simulink model "flightControlSystem"  (R2024a)
settings: Solver=ode3  StartTime=0  StopTime=TFinal  FixedStep=Ts  RelTol=1e-3  EnableMultiTasking=on
model workspace (MAT data in the model file):
  CIRCLE_PTS = [19 19 19]
  ZEROS = [0 0 0 0 0 0 0 0 0 0 0 0 ... (1444 elements, 38x38)]
undefined symbols (not defined in the file): codertarget, Controller, DiscIntNeverNeededParam, Discrete, Estimator, g, gray, init, Sensors, Time, Ts, var_acc_angle_N, var_bias_gyr_N, var_gyro_p_N, Vehicle
libraries: simulink x38, slpidlib x4, ctrlSharedLib x4, sharedtransform x3, visiontextngfix x1, parrotlib x1
(part 3 of 3)

== matlab function flightControlSystem/Image Processing System/Subsystem2/Subsystem1/scan_range ==
  data: result output; u input; startX input; startY input; endX input; endY input; isScanning input
function result = scan_range(u, startX, startY, endX, endY, isScanning)

currentX = 1;
currentY = 2;
movementSpeed = 0;
redLinePresence = u(60, 80);

persistent previousEndlessX;
persistent previousEndlessY;

if isScanning
    if redLinePresence == 1  % ------ inside red-line ------
    
        maxDistance = 0;
        count = 0;

        endlessX = [0 0];
        endlessY = [0 0];
        timeCount = [0 0];

        isEndless = false;
        endlessIndex = 0;
        
        edgeDir = edgeCount(startX, startY);
        xi = startX;  yi = startY; direction = 1;
        
        if edgeDir == 1 || edgeDir == 4
            direction = -1;
        end
        
        while xi ~= endX || yi ~= endY
            distance = drawLine(60, 80, xi, yi, u, 0);

            if distance == 0 % if endless

                if ~isEndless
                    isEndless = true;
                    endlessIndex = endlessIndex + 1;
                end
                if endlessIndex > 2
                    break;
                end
                
                endlessX(endlessIndex) = endlessX(endlessIndex) + xi;
                endlessY(endlessIndex) = endlessY(endlessIndex) + yi;
                timeCount(endlessIndex) = timeCount(endlessIndex) + 1;

            else
                isEndless = false;
                if distance > maxDistance
                    maxDistance = distance;
                    currentX = xi; 
                    currentY = yi;
                    count = 1;
                end
            end

            % Iteration
            edgeDir = edgeCount(xi, yi);
            if edgeDir == 1 || edgeDir == 3
                yi = yi + direction;
            else
                xi = xi + direction;
            end
            if xi < 1
                yi = 159; xi = 1; direction = -1;
            elseif xi > 120
                xi = 120; yi = 2; direction = 1;
            elseif yi < 1
                yi = 1; xi = 2; direction = 1;
            elseif yi > 160
                yi = 160; xi = 119; direction = -1;
            end
        end % while end

        if endlessIndex == 1 % ---------- 1 endless ------------
            currentX = endlessX(1);
            currentY = endlessY(1);
            count = timeCount(1);

            currentX = round(currentX / count);
            currentY = round(currentY / count);
            [currentX, currentY] = closestEdge(currentX, currentY);

            previousEndlessX = 60 + (60 - currentX) + 1;
            previousEndlessY = 80 + (80 - currentY) + 1;

        elseif endlessIndex == 2 % ---------- 2 endless ------------
            
            if isempty(previousEndlessX)
                currentX = endlessX(1);
                currentY = endlessY(1);
                count = timeCount(1);
    
                currentX = round(currentX / count);
                currentY = round(currentY / count);
                [currentX, currentY] = closestEdge(currentX, currentY);
    
                previousEndlessX = 60 + (60 - currentX) + 1;
                previousEndlessY = 80 + (80 - currentY) + 1;
            else
                midPoints = [0 0; 0 0];
                for i = 1:2
                    x = endlessX(i);
                    y = endlessY(i);
                    t = timeCount(i);

                    x = round(x / t);
                    y = round(y / t);
                    
                    [x, y] = closestEdge(x, y);
                    
                    midPoints(i, 1) = x;
                    midPoints(i, 2) = y;
                end

                diff1X = previousEndlessX - midPoints(1, 1);
                diff1Y = previousEndlessY - midPoints(1, 2);
                diff2X = previousEndlessX - midPoints(2, 1);
                diff2Y = previousEndlessY - midPoints(2, 2);
                distance1 = sqrt(diff1X * diff1X + diff1Y * diff1Y);
                distance2 = sqrt(diff2X * diff2X + diff2Y * diff2Y);

                if distance1 > distance2
                    currentX = midPoints(1, 1);
                    currentY = midPoints(1, 2);
                else
                    currentX = midPoints(2, 1);
                    currentY = midPoints(2, 2);
                end
                
                previousEndlessX = 60 + (60 - currentX) + 1;
                previousEndlessY = 80 + (80 - currentY) + 1;
                
            end
        else % ---------- NO endless ------------
            movementSpeed = maxDistance;
        end

    else % ----------------- outside red line ----------------------
        startX = 2; startY = 1;
        endX = 1; endY = 1;
        
        MAX_DISTANCE = 100;
        minDistance = MAX_DISTANCE;
        edgeDir = edgeCount(startX, startY);
        xi = startX;  yi = startY; direction = 1;
        if edgeDir == 1 || edgeDir == 4
            direction = -1;
        end
        
        while xi ~= endX || yi ~= endY
            distance = drawLine(60, 80, xi, yi, u, 1);
    
            if distance > 0 && distance < minDistance
                minDistance = distance;
                currentX = xi;
                currentY = yi;
            end
    
            % Iteration
            edgeDir = edgeCount(xi, yi);
            if edgeDir == 1 || edgeDir == 3
                yi = yi + direction;
            else
                xi = xi + direction;
            end
            if xi < 1
                yi = 159; xi = 1; direction = -1;
            elseif xi > 120
                xi = 120; yi = 2; direction = 1;
            elseif yi < 1
                yi = 1; xi = 2; direction = 1;
            elseif yi > 160
                yi = 160; xi = 119; direction = -1;
            end
        end % while
        
        movementSpeed = 100;
        if minDistance < 60
            movementSpeed = 60;
        end
    end % if redline end

end % isScanning

result = [currentX, currentY, movementSpeed];

end % function end

== matlab function flightControlSystem/Image Processing System/Subsystem2/Subsystem1/check_last_way ==
  data: imageData input; scanStatus output; isRedPixel output; lastPosition input; distanceThreshold input; movement output
function [scanStatus, isRedPixel, movement] = fcn(imageData, lastPosition, distanceThreshold)

lastX = lastPosition(1);
lastY = lastPosition(2);

isRedPixel = imageData(60, 80);
pixelCompare = ~isRedPixel;

scanStatus = 0;
targetX = 1;
targetY = 1;
motionSpeed = 0;

if lastX == 0 || lastY == 0
    scanStatus = 1;
else 
    if imageData(lastX, lastY) == 1 

        % Endless continuation
        [midPointX, midPointY] = middle_point_of_endless_line(imageData, lastX, lastY);

        targetX = lastX + midPointX;
        targetY = lastY + midPointY;
        
        % Ensure the target position is within bounds
        if targetY > 160
            if targetX == 120 
                targetX = 120 - mod(targetY, 160);
            elseif targetX == 1 
                targetX = mod(targetY, 160);
            end
            targetY = 160;
            
        elseif targetY < 1
            if targetX == 120 
                targetX = 120 - abs(targetY);
            elseif targetX == 1 
                targetX = abs(targetY); 
            end
            targetY = 1;
            
        elseif targetX < 1
            if targetY == 160
                targetY = 160 - abs(targetX);
            elseif targetY == 1
                targetY = abs(targetX);
            end
            targetX = 1;
            
        elseif targetX > 120
            if targetY == 160
                targetY = 160 - (targetX - 120);
            elseif targetY == 1
                targetY = targetX - 120;
            end
            targetX = 120;
        end

        motionSpeed = 100;

    else 
        
        % Endless disappearance
        if isRedPixel
            distance = drawLine(60, 80, lastX, lastY, imageData, pixelCompare);
            if distance < distanceThreshold
                scanStatus = 1;
                motionSpeed = 0;
            else
                motionSpeed = distance;
            end
            
            targetX = lastX;
            targetY = lastY;
        else
            scanStatus = 1;
            targetX = lastX;
            targetY = lastY;
            motionSpeed = 40;
        end

    end
end
movement = [targetX, targetY, motionSpeed];

end % function end

function [midX, midY] = middle_point_of_endless_line(imageData, x, y)

edgeValue = edgeCount(x, y);

if edgeValue == 1 || edgeValue == 3

    % Move to the right
    iterY = y;
    iterX = x;
    direction = 1;
    axisFlag = 0; % 0:y   1:x
    distance = 0;

    while imageData(iterX, iterY) == 1
        if axisFlag == 0
            iterY = iterY + direction;
        else
            iterX = iterX + direction;
        end
        distance = distance + 1;
        
        if iterY > 160
            iterY = 160;
            axisFlag = 1;
            if iterX == 120
                direction = -1;
            elseif iterX == 1
                direction = 1;
            end
        end
        if iterX < 1
            break;
        elseif iterX > 120
            break;
        end
    end
    rightDist = distance;

    % Move to the left
    iterY = y;
    iterX = x;
    direction = -1;
    axisFlag = 0; % 0:y   1:x
    distance = 0;
    
    while imageData(iterX, iterY) == 1
        if axisFlag == 0
            iterY = iterY + direction;
        else
            iterX = iterX + direction;
        end
        distance = distance + 1;

        if iterY < 1
            iterY = 1;
            axisFlag = 1;
            if iterX == 120
                direction = -1;
            elseif iterX == 1
                direction = 1;
            end
        end
        if iterX < 1
            break
        elseif iterX > 120
            break
        end
    end
    leftDist = distance;
    
    
    midX = 0;
    diff = rightDist - leftDist;
    
    if abs(diff) >= 7 && abs(diff) < 25
        midY = round(diff/2);
    else
        midY = 0;
    end

else % Move up or down
    % Move up
    iterX = x;
    iterY = y;
    direction = -1;
    axisFlag = 1; % 0:y   1:x
    distance = 0;
    while imageData(iterX, iterY) == 1
        if axisFlag == 0
            iterY = iterY + direction;
        else
            iterX = iterX + direction;
        end
        distance = distance + 1;

        if iterX < 1
            iterX = 1;
            axisFlag = 0;
            if iterY == 1
                direction = 1;
            elseif iterY == 160
                direction = -1;
            end
        end
        if iterY > 160
            break
        elseif iterY < 1
            break
        end
    end
    upDist = distance;

    % Move down
    iterX = x;
    iterY = y;
    direction = 1;
    axisFlag = 1; % 0:y   1:x
    distance = 0;
    while imageData(iterX, iterY) == 1
        if axisFlag == 0
            iterY = iterY + direction;
        else
            iterX = iterX + direction;
        end
        distance = distance + 1;
        if iterX > 120
            axisFlag = 0;
            iterX = 120;
            if iterY == 1
                direction = 1;
            elseif iterY == 160
                direction = -1;
            end
        end
        if iterY > 160
            break;
        elseif iterY < 1
            break;
        end
    end
    downDist = distance;

    diff = downDist - upDist;

    midY = 0;
    if abs(diff) >= 7 && abs(diff) < 25
        midX = round(diff/2);
    else
        midX = 0;
    end
end

end

== matlab function flightControlSystem/Image Processing System/circle_detection ==
  data: template input; direction output; image input; isDetected output
function [direction,isDetected ] = identify_landing(template,image)

persistent landingStatus;
if isempty(landingStatus)
    landingStatus = 0;
end

isDetected = 0;
direction = [0 0 0];
landingFlag = 0;

if landingStatus == 1
    direction = [0 0 1];
    isDetected = 1;

else
    [pixelCount, centerX, centerY] = detect_circle(image, template);
    
    if pixelCount >= 1350
        isDetected = 1;
        centerX = centerX + 19;
        centerY = centerY + 19;
    
        if centerX > 120
            centerX = 120;
        end
        if centerY > 160
            centerY = 160;
        end
        
        deltaX = round(60 - centerX);
        deltaY = round(centerY - 80);
        
        distance = sqrt(deltaX * deltaX + deltaY * deltaY);
    
        fprintf(' ##Landing..!\n');
    
        if distance < 15
            landingFlag = 1;
            landingStatus = 1;
        end
        directionX = deltaX / 130000;
        directionY = deltaY / 130000;
        direction = [directionX directionY landingFlag];
    end

end

end

function [pixelCount, coordX, coordY] = detect_circle(image, template)

% pixelCount: sum of number of pixels
% coordX: row coordinate of image
% coordY: column coordinate of image

[templateRows, templateCols] = size(template);
rows = 120;  
cols = 160;

pixelCount = 0;
coordX = 0;
coordY = 0;

for i = 1:(rows - templateRows)
    for j = 1:(cols - templateCols)
        section = image(i:i+templateRows-1, j:j+templateCols-1);
        matchCount = sum(~xor(section, template), 'all');
        if matchCount > pixelCount
            pixelCount = matchCount;
            coordX = i;
            coordY = j;
        end
    end

end
end

== matlab function flightControlSystem/Image Processing System/Subsystem2/Display ==
  data: r input; R output; g input; b input; way_x input; way_y input; G output; B output
function [R, G, B] = drawArrow(r, g, b, way_x, way_y)
% This function draws arrows on the image at specific coordinates.


%circle draw
function [r, g, b] = drawCircle(r, g, b, center_x, center_y, radius, color)
    % Draw a circle on the image with the specified center and radius

    [rows, cols] = size(r);

    % Check that the center is within the image boundaries
    if center_x < 1 || center_x > rows || center_y < 1 || center_y > cols
        error('Center point is outside the image boundaries.');
    end
    
    % Generate a grid of coordinates
    [X, Y] = meshgrid(1:cols, 1:rows);
    
    % Calculate the distance of each point from the center
    distances = sqrt((X - center_y).^2 + (Y - center_x).^2);
    
    % Create a binary mask for the circle
    circle_mask = distances <= radius;
    
    % Apply the color to the circle mask
    r(circle_mask) = color(1);
    g(circle_mask) = color(2);
    b(circle_mask) = color(3);
end




% Helper function to draw a line with a specific color
function [r, g, b] = drawLine(r, g, b, x1, y1, x2, y2, color)
    swapped = 0;
    if abs(y2 - y1) > abs(x2 - x1)
        swapped = 1;
        [x1, y1] = deal(y1, x1);
        [x2, y2] = deal(y2, x2);
        xk = 1; yk = 1;
        if x2 < x1, xk = -1; end
        if y2 < y1, yk = -1; end
    else
        xk = -1; yk = -1;
        if x2 > x1, xk = 1; end
        if y2 > y1, yk = 1; end
    end
    dy = abs(y2 - y1);
    dx = abs(x2 - x1);
    m = 2 * dy;
    slope_error = m - 2 * dx;
    y = y1;
    for x = x1:xk:x2
        if swapped == 1
            if y >= 1 && y <= size(r, 1) && x >= 1 && x <= size(r, 2)
                r(y, x) = color(1);
                g(y, x) = color(2);
                b(y, x) = color(3);
            end
        else
            if x >= 1 && x <= size(r, 1) && y >= 1 && y <= size(r, 2)
                r(x, y) = color(1);
                g(x, y) = color(2);
                b(x, y) = color(3);
            end
        end
        slope_error = slope_error + m;
        if slope_error > 0
            y = y + yk;
            slope_error = slope_error - 2 * dx;
        end
    end
end

% Helper function to draw an arrowhead at the end of the line
function [r, g, b] = drawArrowhead(r, g, b, x1, y1, x2, y2, color)
    % Calculate the angle of the line
    angle = atan2(y2 - y1, x2 - x1);
    % Arrowhead parameters
    arrowSize = 10;
    arrowAngle = pi / 6; % 30 degrees
    % Calculate the points of the arrowhead
    xLeft = x2 - arrowSize * cos(angle - arrowAngle);
    yLeft = y2 - arrowSize * sin(angle - arrowAngle);
    xRight = x2 - arrowSize * cos(angle + arrowAngle);
    yRight = y2 - arrowSize * sin(angle + arrowAngle);
    % Draw the arrowhead
    [r,g,b] = drawLine(r, g, b, x2, y2, xLeft, yLeft, color);
    [r,g,b] = drawLine(r, g, b, x2, y2, xRight, yRight, color);
end

% Set the pixel at (60, 80) to green
if 60 >= 1 && 60 <= size(r, 1) && 80 >= 1 && 80 <= size(r, 2)
    r(60, 80) = 0; 
    g(60, 80) = 255; 
    b(60, 80) = 0; % Green
    color=[0,115,0];
    g=drawCircle(r,g,b,60,80,20,color);
end

% Draw a green arrow from (60, 80) to (way_x, way_y)
if way_x >= 1 && way_y >= 1 && way_x <= size(r, 1) && way_y <= size(r, 2)
    color = [0, 0, 240]; % Green
    [r,g,b] = drawLine(r, g, b, 60, 80, way_x, way_y, color);
    [r,g,b] = drawArrowhead(r, g, b, 60, 80, way_x, way_y, color);
end


% Return the modified color channels
R = r;
G = g;
B = b;
end

== matlab function flightControlSystem/Image Processing System/Subsystem2/Subsystem1/Data_Editor ==
  data: destination input; outputWay output; isRed input; previousXY input; currentX output; currentY output
function [outputWay, currentX, currentY] = fcn(destination, isRed, previousXY)

xCoord = destination(1);
yCoord = destination(2);
velocity = destination(3);

if isRed
    X = xCoord;   
    Y = yCoord;
    currentX = xCoord;  
    currentY = yCoord;
else
    X = xCoord;  
    Y = yCoord; 
    currentX = previousXY(1);  
    currentY = previousXY(2);
end

outputWay = [X Y velocity];

%fprintf('X = %f | Y = %f\n', currentX, currentY);
end

== matlab function flightControlSystem/Control System/Controller/Position Controller/Position error transformation (Earth to Body frame) ==
  data: yaw input; xy_err_earth input; xy_err_body output
function xy_err_body = fcn(yaw,xy_err_earth)

transformation = [cos(yaw), sin(yaw); -sin(yaw),  cos(yaw)];
xy_err_body = transformation * xy_err_earth;


end

== matlab function flightControlSystem/Image Processing System/Subsystem2/Subsystem1/speed_Manage ==
  data: inputWay input; adjustedX output; adjustedY output
function [adjustedX, adjustedY] = fcn(inputWay)

xCoord = inputWay(1);
yCoord = inputWay(2);
velocity = inputWay(3);

if velocity == 100
    velocity = 200;
elseif velocity < 60
    velocity = 60;
end

adjustedX = (60 - xCoord) / 10000000 * velocity;
adjustedY = (yCoord - 80) / 10000000 * velocity;

%fprintf(' --- speed: %f | ', velocity); fprintf('vectors: X=%.5f | Y=%.5f\n', adjustedX, adjustedY);

end

== matlab function flightControlSystem/Image Processing System/Subsystem2/opposite_way ==
  data: newX output; currentPosition input; newY output
function [newX, newY] = calculate_opposite_coordinates(currentPosition)

    x = currentPosition(1);
    y = currentPosition(2);
    
    if x == 0 || y == 0
        newX = 0;
        newY = 0;
    else
        newX = 60 + (60 - x) + 1;
        newY = 80 + (80 - y) + 1;
    end

    %fprintf('opposite: %.0f %.0f -> %.0f %.0f\n', x, y, newX, newY);
end

== matlab function flightControlSystem/Image Processing System/Subsystem2/Subsystem1/center_vector_x ==
  data: image input; slide_x output
function slide_x = compute_slide_x(image)
    row_center = 60; 
    col_center = 80;
    left_x = 0;
    right_x = 0;
    middle_pixel = image(row_center, col_center);
    compare_pixel = ~middle_pixel;
    
    % Look left for the line
    for i = col_center:-1:60
        if image(row_center, i) == compare_pixel
            left_x = i;
            break
        end
    end
    
    % Look right for the line
    for i = col_center:100
        if image(row_center, i) == compare_pixel
            right_x = i;
            break
        end
    end

    slide_x = 0;
    if left_x ~= 0 && right_x ~= 0 % in line
        if middle_pixel == 1
            length_right = right_x - col_center;  % length right 
            length_left = col_center - left_x;   % length left
            diff = length_right - length_left;
            slide_x = determine_speed(diff) * 20;
        end
    end
end

function speed = determine_speed(diff)
    % Determine speed based on the difference diff
    if diff > 0
        if diff < 1
            speed = 0.000001;
        elseif diff < 5
            speed = 0.000002;
        elseif diff < 10
            speed = 0.000003;
        elseif diff < 15
            speed = 0.000004;
        elseif diff < 20
            speed = 0.000005;
        else
            speed = 0.000006;
        end
    else
        if diff < -20
            speed = -0.000006;
        elseif diff < -15
            speed = -0.000005;
        elseif diff < -10
            speed = -0.000004;
        elseif diff < -5
            speed = -0.000003;
        elseif diff < -1
            speed = -0.000002;
        else
            speed = -0.000001;
        end
    end
end

== matlab function flightControlSystem/Image Processing System/Subsystem2/Subsystem1/range_points ==
  data: newX input; startX output; newY input; reference input; startY output; endX output; endY output
function [startX, startY, endX, endY] = get_range_points(newX, newY, reference)

% startX, startY are the coordinates on the left
% endX, endY are the coordinates on the right
% according to the center-to-edge vector.ca

edgeDirection = edgeCount(newX, newY);

if edgeDirection == 1
    startY = newY - reference;
    if startY < 1
        startX = newX - startY;
        startY = 1;
    else
        startX = newX;
    end

    endY = newY + reference;
    if endY > 160
        endX = endY - 160;
        endY = 160;
    else
        endX = newX;
    end
elseif edgeDirection == 2
    startX = newX + reference;
    if startX > 120
        startY = startX - 120;
        startX = 120;
    else
        startY = newY;
    end

    endX = newX - reference;
    if endX < 1
        endY = abs(endX) + 1;
        endX = 1;
    else
        endY = newY;
    end
elseif edgeDirection == 4
    startX = newX - reference;
    if startX < 1
        startY = 160 + startX;
        startX = 1;
    else
        startY = 160;
    end

    endX = newX + reference;
    if endX > 120
        endY = 160 - (endX - 120);
        endX = 120;
    else
        endY = newY;
    end
elseif edgeDirection == 3
    startY = newY + reference;
    if startY > 160
        startX = 120 - (startY - 160);
        startY = 160;
    else
        startX = newX;
    end

    endY = newY - reference;
    if endY < 1
        endX = 120 + endY;
        endY = 1;
    else
        endX = newX;
    end
else
    startX = 1; startY = 1;
    endX = 1; endY = 2;
end

%fprintf('range_points: %.0f-%.0f  to  %.0f-%.0f\n', startX, startY, endX, endY);

end

== stateflow chart flightControlSystem/Control System/Path Planning/Subsystem/Chart ==
  state hover
    xOut = 0;
    yOut = 0;
    zOut = -1.1;
  state go
    xOut = xOut + xin;
    yOut = yOut + yin;
    zOut = -1.1;
  state land
    zOut = 0.6;
    xOut = xOut;
    yOut = yOut;
  state Final_landing
    zOut = 0;
    xOut = xOut;
    yOut = yOut;
  (default) -> hover
  go -> land : [land==1]
  hover -> go : [after(4, sec)]
  land -> Final_landing : [land==1 && zEsti==0.6]
  data: zEsti input; xOut output; yOut output; zOut output; yin input; xin input; land input

== matlab function flightControlSystem/Control System/Path Planning/Subsystem/path_analyzer ==
  data: coordX output; inputVector input; coordY output; isLanding output
function [coordX, coordY, isLanding] = fcn(inputVector)

coordX = inputVector(1);
coordY = inputVector(2);
isLanding = inputVector(3);

end
